simulink subsystem "Sound"  (R2023b)
settings: Solver=VariableStepAuto  StartTime=0.0  StopTime=10.0  RelTol=1e-3
libraries: dspsnks4 x1, audiosources x1
settings Model: Creator=diego  LastModifiedBy=Greg

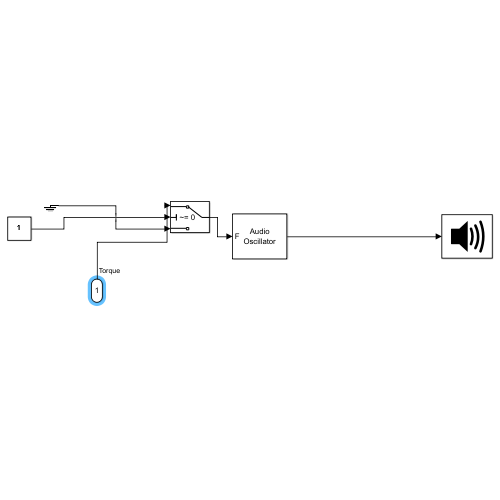
[thumbnail: Simulink's stored preview of the top-level diagram]
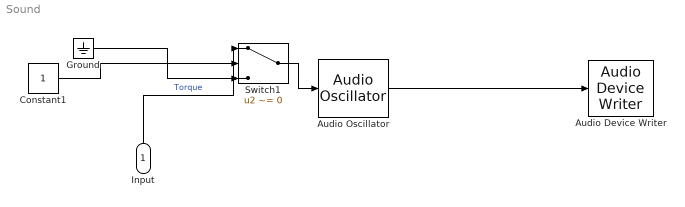
== system Sound ==
  Input : Inport
  Audio Device Writer : dspsnks4/Audio Device Writer  Driver=DirectSound  Device=Default  InheritSampleRate=on  SampleRate=44100  BitDepth=16-bit integer  BufferSize=4096  NumBuffers=10  DefaultOutputChannelMapping=on  OutputChannelMapping=1:2  OutputNumUnderrunSamples=off  DriverIdx=1  DeviceWarnFlag=''
  Audio Oscillator : audiosources/Audio Oscillator  FrequencyPort=on  Frequency=100  AmplitudePort=off  Amplitude=1  DCOffsetPort=off  PhaseOffset=0  DCOffset=0  WidthPort=off  Width=1  DutyCyclePort=off  DutyCycle=0.5  SampsPerFrame=512  Fs=44100  OutputDataType=double  SimulateUsing=Code generation
      settings: SignalType=square
  Constant1 : Constant  SampleTime=-1
  Ground : Ground
  Switch1 : Switch  Criteria=u2 ~= 0  SaturateOnIntegerOverflow=off  InputSameDT=off
  wires:
  Switch1/1 -> Audio Oscillator/1
  Constant1/1 -> Switch1/2
  Ground/1 -> Switch1/3
  Audio Oscillator/1 -> Audio Device Writer/1
  Input/1 -> Switch1/1  "Torque"
